simulink model "house_dynamics"  (R2015b)
settings: Solver=VariableStepAuto  StartTime=0.0  StopTime=len_sim*3600  RelTol=1e-3
values from neighbouring files (symbols this model uses):
  amb_CO = xlsread(filename,'Sheet1','X33')    [main_code.m]
  amb_CO2 = xlsread(filename,'Sheet1','X32')    [main_code.m]
  amb_PM = xlsread(filename,'Sheet1','X34')    [main_code.m]
  Cp_air = xlsread(filename,'Sheet1','X29')    [main_code.m]
  h_wall = xlsread(filename,'Sheet1','I30')    [main_code.m]
  k_door = door(1)    [main_code.m]
  k_floor = floor(1)    [main_code.m]
  k_roof_1 = roof_1(1)    [main_code.m]
  k_roof_2 = roof_2(1)    [main_code.m]
  k_roof_3 = roof_3(1)    [main_code.m]
  k_roof_4 = roof_4(1)    [main_code.m]
  k_roof_5 = roof_5(1)    [main_code.m]
  k_wall_a_1 = wall_a_1(1)    [main_code.m]
  k_wall_a_2 = wall_a_2(1)    [main_code.m]
  k_wall_a_3 = wall_a_3(1)    [main_code.m]
  k_wall_a_4 = wall_a_4(1)    [main_code.m]
  k_wall_a_5 = wall_a_5(1)    [main_code.m]
  k_wall_b_1 = wall_b_1(1)    [main_code.m]
  k_wall_b_2 = wall_b_2(1)    [main_code.m]
  k_wall_b_3 = wall_b_3(1)    [main_code.m]
  k_wall_b_4 = wall_b_4(1)    [main_code.m]
  k_wall_b_5 = wall_b_5(1)    [main_code.m]
  k_wall_c_1 = wall_c_1(1)    [main_code.m]
  k_wall_c_2 = wall_c_2(1)    [main_code.m]
  k_wall_c_4 = wall_c_4(1)    [main_code.m]
  k_wall_c_5 = wall_c_5(1)    [main_code.m]
  k_wall_d_1 = wall_d_1(1)    [main_code.m]
  k_wall_d_2 = wall_d_2(1)    [main_code.m]
  k_wall_d_3 = wall_d_3(1)    [main_code.m]
  k_wall_d_4 = wall_d_4(1)    [main_code.m]
  k_wall_d_5 = wall_d_5(1)    [main_code.m]
  k_window = window(1)    [main_code.m]
  l_wall = xlsread(filename,'Sheet1','I29')    [main_code.m]
  roof_c1 = alpha_roof_1/(t_roof_1*t_roof_1)    [main_code.m]
  roof_c2 = alpha_roof_2/(t_roof_2*t_roof_2)    [main_code.m]
  roof_c3 = alpha_roof_3/(t_roof_3*t_roof_3)    [main_code.m]
  roof_c4 = alpha_roof_4/(t_roof_4*t_roof_4)    [main_code.m]
  roof_c5 = alpha_roof_5/(t_roof_5*t_roof_5)    [main_code.m]
  roof_p1 = 4*t_roof_1*hb/k_roof_1    [main_code.m]
  roof_p2 = 4*t_roof_5*hinf/k_roof_5    [main_code.m]
  t_door = door(5)    [main_code.m]
  t_floor = floor(5)    [main_code.m]
  t_roof_1 = roof_1(5)    [main_code.m]
  t_roof_2 = roof_2(5)    [main_code.m]
  t_roof_3 = roof_3(5)    [main_code.m]
  t_roof_4 = roof_4(5)    [main_code.m]
  t_roof_5 = roof_5(5)    [main_code.m]
  t_wall_a_1 = wall_a_1(5)    [main_code.m]
  t_wall_a_2 = wall_a_2(5)    [main_code.m]
  t_wall_a_3 = wall_a_3(5)    [main_code.m]
  t_wall_a_4 = wall_a_4(5)    [main_code.m]
  t_wall_a_5 = wall_a_5(5)    [main_code.m]
  t_wall_b_1 = wall_b_1(5)    [main_code.m]
  t_wall_b_2 = wall_b_2(5)    [main_code.m]
  t_wall_b_3 = wall_b_3(5)    [main_code.m]
  t_wall_b_4 = wall_b_4(5)    [main_code.m]
  t_wall_b_5 = wall_b_5(5)    [main_code.m]
  t_wall_c_1 = wall_c_1(5)    [main_code.m]
  t_wall_c_2 = wall_c_2(5)    [main_code.m]
  t_wall_c_4 = wall_c_4(5)    [main_code.m]
  t_wall_c_5 = wall_c_5(5)    [main_code.m]
  t_wall_d_1 = wall_d_1(5)    [main_code.m]
  t_wall_d_2 = wall_d_2(5)    [main_code.m]
  t_wall_d_3 = wall_d_3(5)    [main_code.m]
  t_wall_d_4 = wall_d_4(5)    [main_code.m]
  t_wall_d_5 = wall_d_5(5)    [main_code.m]
  t_window = window(5)    [main_code.m]
  To = initial_room_temp    [main_code.m]
  w_wall = xlsread(filename,'Sheet1','I28')    [main_code.m]
settings Model: Creator=Sahil Desai  LastModifiedBy=Sahil Desai

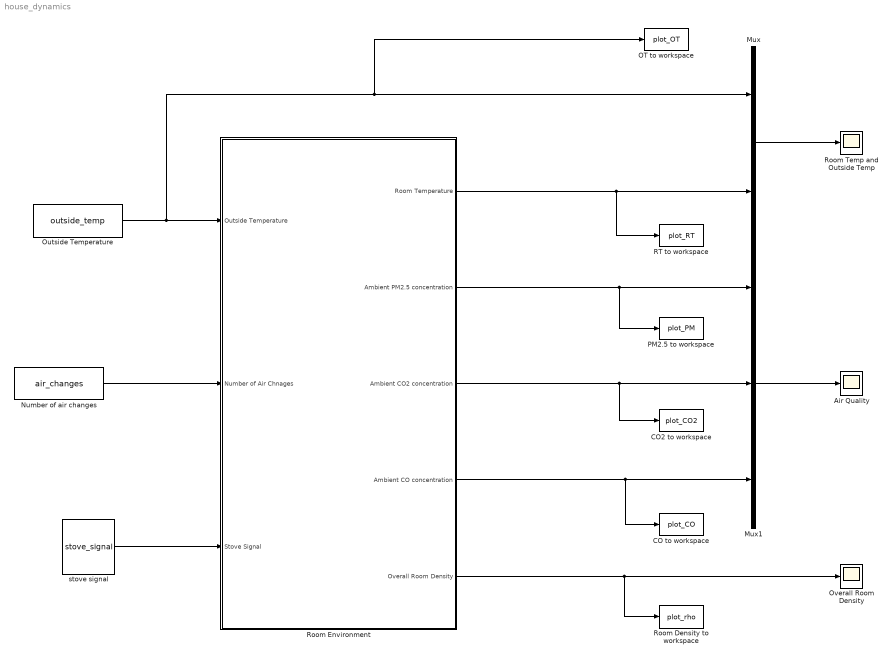
== system house_dynamics ==
  Air Quality : Scope
  CO to workspace : ToWorkspace  VariableName=plot_CO  SampleTime=-1
  CO2 to workspace : ToWorkspace  VariableName=plot_CO2  SampleTime=-1
  Mux : Mux  Inputs=2
  Mux1 : Mux  Inputs=3
  Number of air changes : FromWorkspace  VariableName=air_changes  SampleTime=0
  OT to workspace : ToWorkspace  VariableName=plot_OT  SampleTime=-1
  Outside Temperature : FromWorkspace  VariableName=outside_temp  SampleTime=0
  Overall Room Density : Scope
  PM2.5 to workspace : ToWorkspace  VariableName=plot_PM  SampleTime=-1
  RT to workspace : ToWorkspace  VariableName=plot_RT  SampleTime=-1
  Room Density to workspace : ToWorkspace  VariableName=plot_rho  SampleTime=-1
  Room Environment : Subsystem
  Room Temp and Outside Temp : Scope
  stove signal : FromWorkspace  VariableName=stove_signal  SampleTime=0
  wires:
  Number of air changes/1 -> Room Environment/2(Number of Air Chnages)
  stove signal/1 -> Room Environment/3(Stove Signal)
  Outside Temperature/1 -> OT to workspace/1, Mux/1, Room Environment/1(Outside Temperature)
  Mux/1 -> Room Temp and Outside Temp/1
  Mux1/1 -> Air Quality/1
  Room Environment/5(Overall Room Density) -> Room Density to workspace/1, Overall Room Density/1
  Room Environment/3(Ambient CO2 concentration) -> CO2 to workspace/1, Mux1/2
  Room Environment/2(Ambient PM2.5 concentration) -> PM2.5 to workspace/1, Mux1/1
  Room Environment/4(Ambient CO concentration) -> CO to workspace/1, Mux1/3
  Room Environment/1(Room Temperature) -> RT to workspace/1, Mux/2

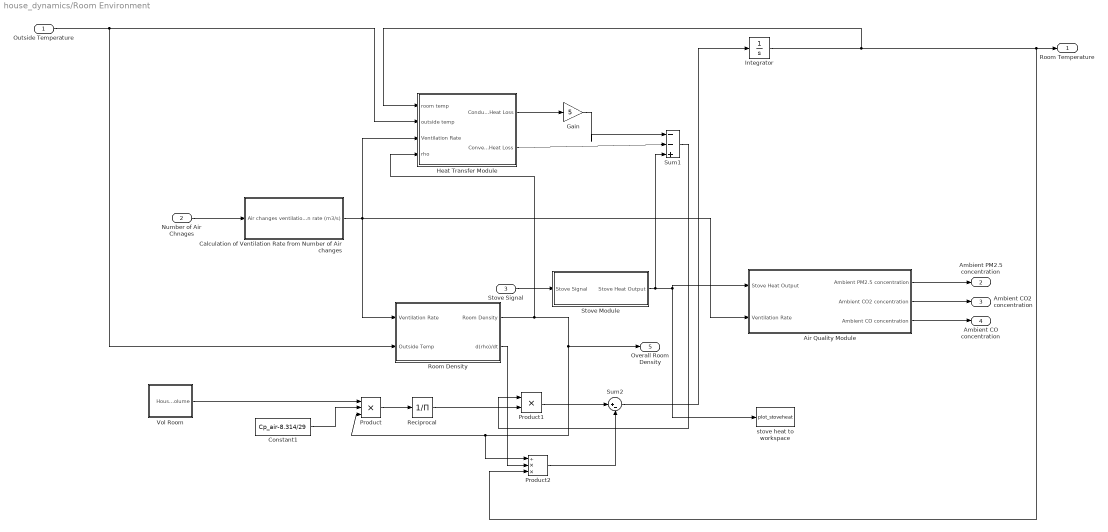
== system house_dynamics/Room Environment ==
  Outside Temperature : Inport
  Number of Air Chnages : Inport  Port=2
  Stove Signal : Inport  Port=3
  Air Quality Module : Subsystem
  Calculation of Ventilation Rate from Number of Air changes : Subsystem
  Constant1 : Constant  Value=Cp_air-8.314/29
  Gain : Gain  Gain=5
  Heat Transfer Module : Subsystem
  Integrator : Integrator  InitialCondition=5
  Product : Product  Inputs=3
  Product1 : Product
  Product2 : Product  Inputs=/**
  Reciprocal : Product  Inputs=/  SaturateOnIntegerOverflow=on  RndMeth=Zero
  Room Density : Subsystem
  Stove Module : Subsystem
  Sum1 : Sum  Inputs=|--+
  Sum2 : Sum  Inputs=|+-
  Vol Room : Subsystem
  stove heat to workspace : ToWorkspace  VariableName=plot_stoveheat  SampleTime=-1
  Room Temperature : Outport
  Ambient PM2.5 concentration : Outport  Port=2
  Ambient CO2 concentration : Outport  Port=3
  Ambient CO concentration : Outport  Port=4
  Overall Room Density : Outport  Port=5
  wires:
  Outside Temperature/1 -> Room Density/2(Outside Temp), Heat Transfer Module/2(outside temp)
  Integrator/1 -> Heat Transfer Module/1(room temp), Room Temperature/1, Product2/3
  Calculation of Ventilation Rate from Number of Air changes/1(ventilation rate (m3/s)) -> Room Density/1(Ventilation Rate), Air Quality Module/2(Ventilation Rate), Heat Transfer Module/3(Ventilation Rate)
  Number of Air Chnages/1 -> Calculation of Ventilation Rate from Number of Air changes/1(Air changes)
  Stove Signal/1 -> Stove Module/1(Stove Signal)
  Room Density/1(Room Density) -> Overall Room Density/1, Product2/1, Product/3, Heat Transfer Module/4(rho)
  Product/1 -> Reciprocal/1
  Reciprocal/1 -> Product1/2
  Sum1/1 -> Product1/1
  Product1/1 -> Sum2/1
  Room Density/2("d(rho)/dt ") -> Product2/2
  Product2/1 -> Sum2/2
  Sum2/1 -> Integrator/1
  Air Quality Module/3(Ambient CO concentration) -> Ambient CO concentration/1
  Air Quality Module/2(Ambient CO2 concentration) -> Ambient CO2 concentration/1
  Air Quality Module/1(Ambient PM2.5 concentration) -> Ambient PM2.5 concentration/1
  Constant1/1 -> Product/2
  Heat Transfer Module/2(Convective Heat Loss) -> Sum1/2
  Heat Transfer Module/1(Conductive Heat Loss) -> Gain/1
  Vol Room/1(House Volume) -> Product/1
  Gain/1 -> Sum1/1
  Stove Module/1(Stove Heat Output) -> stove heat to workspace/1, Air Quality Module/1(Stove Heat Output), Sum1/3

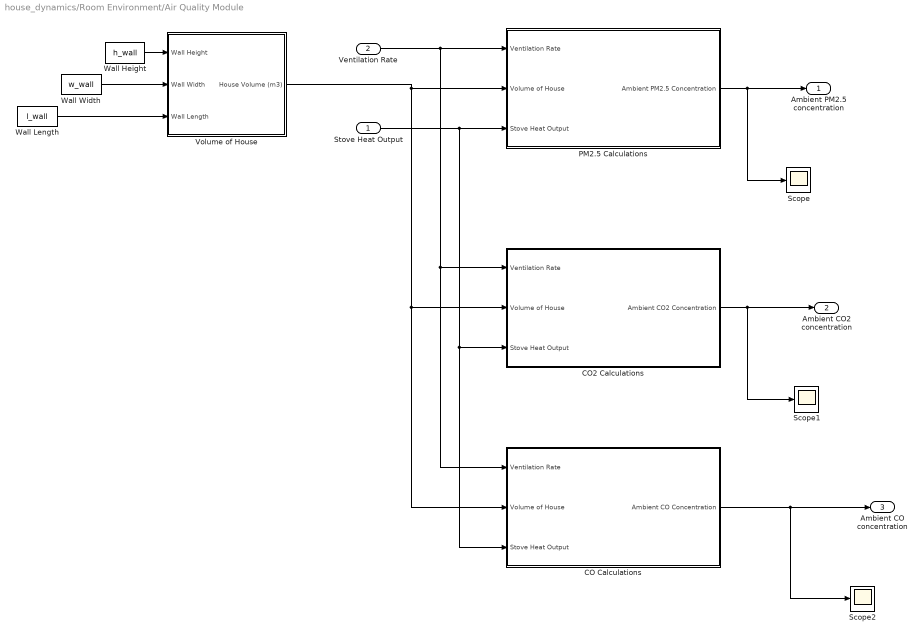
== system house_dynamics/Room Environment/Air Quality Module ==
  Stove Heat Output : Inport
  Ventilation Rate : Inport  Port=2
  CO Calculations : Subsystem
  CO2 Calculations : Subsystem
  PM2.5 Calculations : Subsystem
  Scope : Scope
  Scope1 : Scope
  Scope2 : Scope
  Volume of House : Subsystem  TreatAsAtomicUnit=on
  Wall Height : Constant  Value=h_wall
  Wall Length : Constant  Value=l_wall
  Wall Width : Constant  Value=w_wall
  Ambient PM2.5 concentration : Outport
  Ambient CO2 concentration : Outport  Port=2
  Ambient CO concentration : Outport  Port=3
  wires:
  Ventilation Rate/1 -> CO Calculations/1(Ventilation Rate), CO2 Calculations/1(Ventilation Rate), PM2.5 Calculations/1(Ventilation Rate)
  Stove Heat Output/1 -> CO Calculations/3(Stove Heat Output), CO2 Calculations/3(Stove Heat Output), PM2.5 Calculations/3(Stove Heat Output)
  PM2.5 Calculations/1(Ambient PM2.5 Concentration) -> Scope/1, Ambient PM2.5 concentration/1
  Volume of House/1(House Volume (m3)) -> CO Calculations/2(Volume of House), CO2 Calculations/2(Volume of House), PM2.5 Calculations/2(Volume of House)
  CO2 Calculations/1(Ambient CO2 Concentration) -> Ambient CO2 concentration/1, Scope1/1
  CO Calculations/1(Ambient CO Concentration) -> Scope2/1, Ambient CO concentration/1
  Wall Width/1 -> Volume of House/2(Wall Width)
  Wall Height/1 -> Volume of House/1(Wall Height)
  Wall Length/1 -> Volume of House/3(Wall Length)

== system house_dynamics/Room Environment/Calculation of Ventilation Rate from Number of Air changes ==
  Air changes : Inport
  Gain : Gain  Gain=1/3600
  Product1 : Product
  Volume of House : Subsystem  TreatAsAtomicUnit=on
  Wall Height : Constant  Value=h_wall
  Wall Length : Constant  Value=l_wall
  Wall Width : Constant  Value=w_wall
  ventilation rate (m3/s) : Outport
  wires:
  Gain/1 -> ventilation rate (m3/s)/1
  Product1/1 -> Gain/1
  Air changes/1 -> Product1/2
  Volume of House/1(House Volume (m3)) -> Product1/1
  Wall Width/1 -> Volume of House/2(Wall Width)
  Wall Height/1 -> Volume of House/1(Wall Height)
  Wall Length/1 -> Volume of House/3(Wall Length)

== system house_dynamics/Room Environment/Heat Transfer Module ==
  room temp : Inport
  outside temp : Inport  Port=2
  Ventilation Rate : Inport  Port=3
  rho : Inport  Port=4
  Conduction Heat Transfer : Subsystem
  Convective Heat Transfer : Subsystem
  Individual Roof Layer Temperatures : Scope
  Mux : Mux  Inputs=5
  Roof Heat Transfer1 : Subsystem
  Conductive Heat Loss : Outport
  Convective Heat Loss : Outport  Port=2
  wires:
  Ventilation Rate/1 -> Convective Heat Transfer/3(Ventilation Rate)
  outside temp/1 -> Roof Heat Transfer1/1(Outside Temperature), Convective Heat Transfer/1(Outside Temp), Conduction Heat Transfer/2(Outside Temperature)
  rho/1 -> Convective Heat Transfer/4(rho)
  room temp/1 -> Roof Heat Transfer1/2(Room Temperature), Convective Heat Transfer/2(room temp), Conduction Heat Transfer/1(Room Temperature)
  Conduction Heat Transfer/1("Conductive Heat Loss ") -> Conductive Heat Loss/1
  Convective Heat Transfer/1(Convective Heat Transfer) -> Convective Heat Loss/1
  Roof Heat Transfer1/5(Roof_T5) -> Mux/5
  Roof Heat Transfer1/4(Roof_T4) -> Mux/4
  Roof Heat Transfer1/3(Roof_T3) -> Mux/3
  Roof Heat Transfer1/2(Roof_T2) -> Mux/2
  Roof Heat Transfer1/1(Roof_T1) -> Mux/1
  Mux/1 -> Individual Roof Layer Temperatures/1

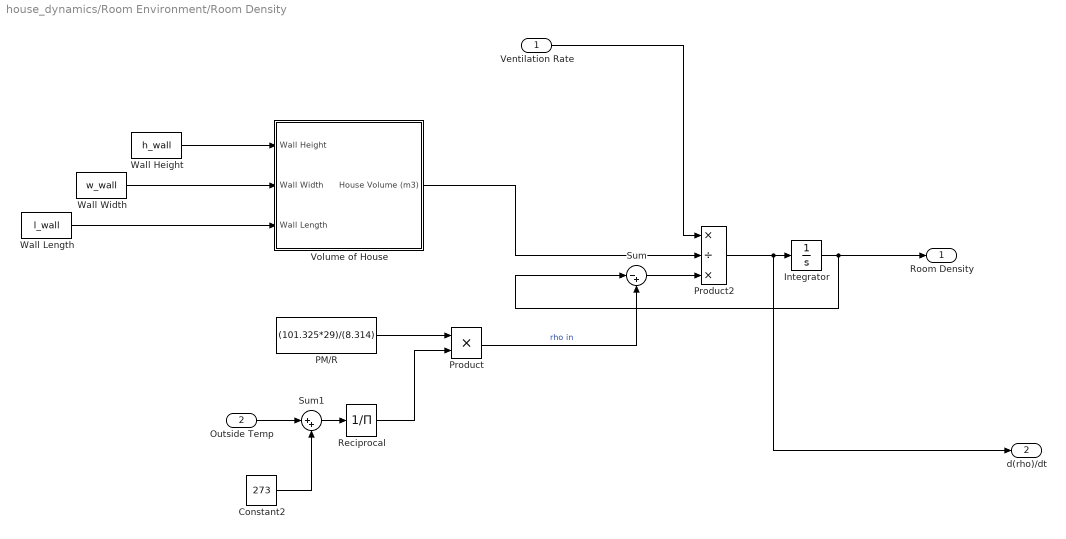
== system house_dynamics/Room Environment/Room Density ==
  Ventilation Rate : Inport
  Outside Temp : Inport  Port=2
  Constant2 : Constant  Value=273
  Integrator : Integrator  InitialCondition=1
  PM/R : Constant  Value=(101.325*29)/(8.314)
  Product : Product
  Product2 : Product  Inputs=*/*
  Reciprocal : Product  Inputs=/  SaturateOnIntegerOverflow=on  RndMeth=Zero
  Sum : Sum  Inputs=|-+
  Sum1 : Sum  Inputs=|++
  Volume of House : Subsystem  TreatAsAtomicUnit=on
  Wall Height : Constant  Value=h_wall
  Wall Length : Constant  Value=l_wall
  Wall Width : Constant  Value=w_wall
  Room Density : Outport
  "d(rho)/dt " : Outport  Port=2
  wires:
  Reciprocal/1 -> Product/2
  PM/R/1 -> Product/1
  Product/1 -> Sum/2  "rho in"
  Sum/1 -> Product2/3
  Product2/1 -> "d(rho)/dt "/1, Integrator/1
  Integrator/1 -> Sum/1, Room Density/1
  Outside Temp/1 -> Sum1/1
  Constant2/1 -> Sum1/2
  Sum1/1 -> Reciprocal/1
  Volume of House/1(House Volume (m3)) -> Product2/2
  Wall Width/1 -> Volume of House/2(Wall Width)
  Wall Height/1 -> Volume of House/1(Wall Height)
  Wall Length/1 -> Volume of House/3(Wall Length)
  Ventilation Rate/1 -> Product2/1

== system house_dynamics/Room Environment/Stove Module ==
  Stove Signal : Inport
  Stove Heat : Subsystem
  Stove Heat Output : Outport
  wires:
  Stove Signal/1 -> Stove Heat/1(Stove Signal)
  Stove Heat/1(Stove Heat Out) -> Stove Heat Output/1

== system house_dynamics/Room Environment/Vol Room ==
  Volume of House : Subsystem  TreatAsAtomicUnit=on
  Wall Height : Constant  Value=h_wall
  Wall Length : Constant  Value=l_wall
  Wall Width : Constant  Value=w_wall
  House Volume : Outport
  wires:
  Volume of House/1(House Volume (m3)) -> House Volume/1
  Wall Width/1 -> Volume of House/2(Wall Width)
  Wall Height/1 -> Volume of House/1(Wall Height)
  Wall Length/1 -> Volume of House/3(Wall Length)

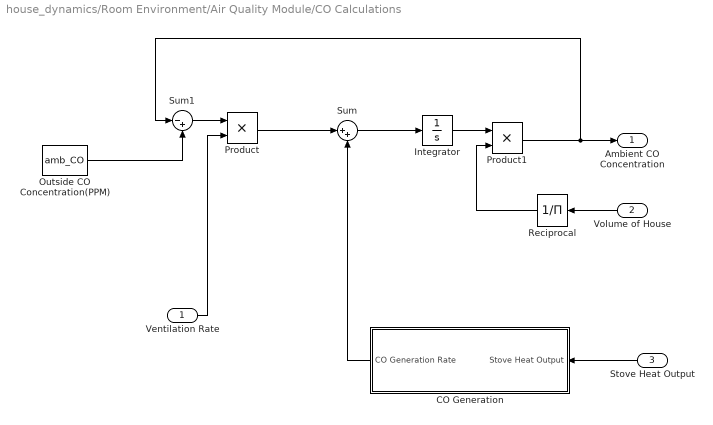
== system house_dynamics/Room Environment/Air Quality Module/CO Calculations ==
  Ventilation Rate : Inport
  Volume of House : Inport  Port=2
  Stove Heat Output : Inport  Port=3
  CO Generation : Subsystem
  Integrator : Integrator  InitialCondition=2
  Outside CO Concentration(PPM) : Constant  Value=amb_CO
  Product : Product
  Product1 : Product
  Reciprocal : Product  Inputs=/  SaturateOnIntegerOverflow=on  RndMeth=Zero
  Sum : Sum  Inputs=|++
  Sum1 : Sum  Inputs=|-+
  Ambient CO Concentration : Outport
  wires:
  Sum/1 -> Integrator/1
  Product/1 -> Sum/1
  CO Generation/1(CO Generation Rate) -> Sum/2
  Stove Heat Output/1 -> CO Generation/1(Stove Heat Output)
  Volume of House/1 -> Reciprocal/1
  Integrator/1 -> Product1/1
  Product1/1 -> Sum1/1, Ambient CO Concentration/1
  Reciprocal/1 -> Product1/2
  Sum1/1 -> Product/1
  Ventilation Rate/1 -> Product/2
  Outside CO Concentration(PPM)/1 -> Sum1/2

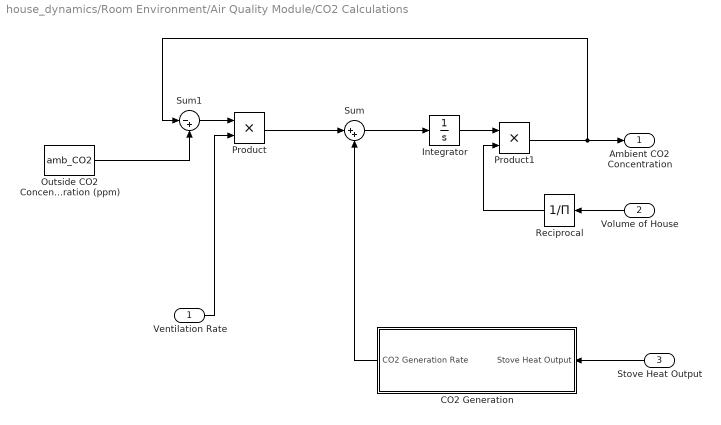
== system house_dynamics/Room Environment/Air Quality Module/CO2 Calculations ==
  Ventilation Rate : Inport
  Volume of House : Inport  Port=2
  Stove Heat Output : Inport  Port=3
  CO2 Generation : Subsystem
  Integrator : Integrator
  Outside CO2 Concentration (ppm) : Constant  Value=amb_CO2
  Product : Product
  Product1 : Product
  Reciprocal : Product  Inputs=/  SaturateOnIntegerOverflow=on  RndMeth=Zero
  Sum : Sum  Inputs=|++
  Sum1 : Sum  Inputs=|-+
  Ambient CO2 Concentration : Outport
  wires:
  Sum/1 -> Integrator/1
  Product/1 -> Sum/1
  CO2 Generation/1(CO2 Generation Rate) -> Sum/2
  Stove Heat Output/1 -> CO2 Generation/1(Stove Heat Output)
  Volume of House/1 -> Reciprocal/1
  Integrator/1 -> Product1/1
  Product1/1 -> Sum1/1, Ambient CO2 Concentration/1
  Reciprocal/1 -> Product1/2
  Sum1/1 -> Product/1
  Ventilation Rate/1 -> Product/2
  Outside CO2 Concentration (ppm)/1 -> Sum1/2

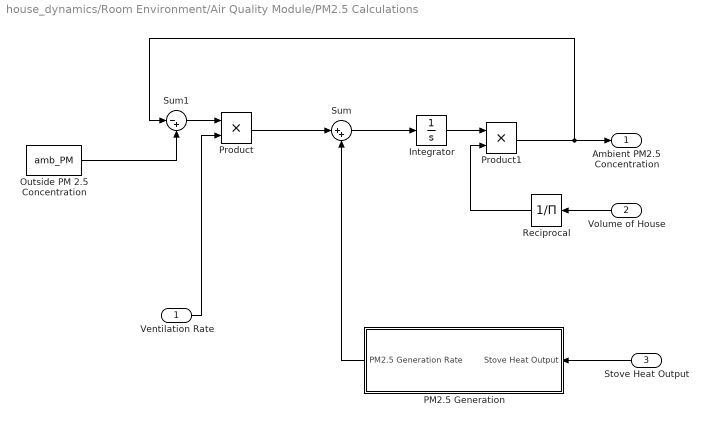
== system house_dynamics/Room Environment/Air Quality Module/PM2.5 Calculations ==
  Ventilation Rate : Inport
  Volume of House : Inport  Port=2
  Stove Heat Output : Inport  Port=3
  Integrator : Integrator
  Outside PM 2.5 Concentration : Constant  Value=amb_PM
  PM2.5 Generation : Subsystem
  Product : Product
  Product1 : Product
  Reciprocal : Product  Inputs=/  SaturateOnIntegerOverflow=on  RndMeth=Zero
  Sum : Sum  Inputs=|++
  Sum1 : Sum  Inputs=|-+
  Ambient PM2.5 Concentration : Outport
  wires:
  Sum/1 -> Integrator/1
  Product/1 -> Sum/1
  PM2.5 Generation/1(PM2.5 Generation Rate) -> Sum/2
  Stove Heat Output/1 -> PM2.5 Generation/1(Stove Heat Output)
  Volume of House/1 -> Reciprocal/1
  Integrator/1 -> Product1/1
  Product1/1 -> Sum1/1, Ambient PM2.5 Concentration/1
  Reciprocal/1 -> Product1/2
  Sum1/1 -> Product/1
  Ventilation Rate/1 -> Product/2
  Outside PM 2.5 Concentration/1 -> Sum1/2

== system house_dynamics/Room Environment/Air Quality Module/Volume of House ==
  Wall Height : Inport
  Wall Width : Inport  Port=2
  Wall Length : Inport  Port=3
  Product : Product  Inputs=3
  House Volume (m3) : Outport
  wires:
  Wall Height/1 -> Product/1
  Wall Width/1 -> Product/2
  Wall Length/1 -> Product/3
  Product/1 -> House Volume (m3)/1

== system house_dynamics/Room Environment/Calculation of Ventilation Rate from Number of Air changes/Volume of House ==
  Wall Height : Inport
  Wall Width : Inport  Port=2
  Wall Length : Inport  Port=3
  Product : Product  Inputs=3
  House Volume (m3) : Outport
  wires:
  Wall Height/1 -> Product/1
  Wall Width/1 -> Product/2
  Wall Length/1 -> Product/3
  Product/1 -> House Volume (m3)/1

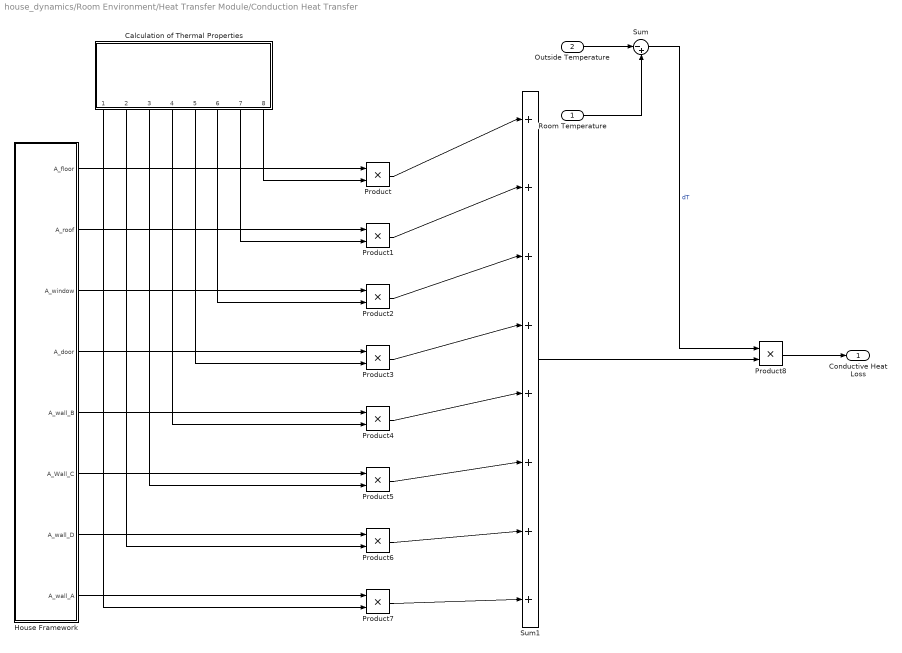
== system house_dynamics/Room Environment/Heat Transfer Module/Conduction Heat Transfer ==
  Room Temperature : Inport
  Outside Temperature : Inport  Port=2
  Calculation of Thermal Properties : Subsystem
  House Framework : Subsystem
  Product{,1..7} (8 alike) : Product  Inputs=**
  Product8 : Product
  Sum : Sum  Inputs=|-+
  Sum1 : Sum  Inputs=|++++++++
  "Conductive Heat Loss " : Outport
  wires:
  House Framework/1(A_floor) -> Product/1
  House Framework/2(A_roof) -> Product1/1
  House Framework/3(A_window) -> Product2/1
  House Framework/4(A_door) -> Product3/1
  House Framework/5(A_wall_B) -> Product4/1
  House Framework/6(A_Wall_C) -> Product5/1
  House Framework/7(A_wall_D) -> Product6/1
  House Framework/8(A_wall_A) -> Product7/1
  Product/1 -> Sum1/1
  Product1/1 -> Sum1/2
  Product2/1 -> Sum1/3
  Product3/1 -> Sum1/4
  Product4/1 -> Sum1/5
  Product5/1 -> Sum1/6
  Product6/1 -> Sum1/7
  Product7/1 -> Sum1/8
  Sum1/1 -> Product8/2
  Sum/1 -> Product8/1  "dT"
  Outside Temperature/1 -> Sum/1
  Room Temperature/1 -> Sum/2
  Product8/1 -> "Conductive Heat Loss "/1
  Calculation of Thermal Properties/8(U_eq_floor) -> Product/2
  Calculation of Thermal Properties/7(U_eq_roof) -> Product1/2
  Calculation of Thermal Properties/6(U_eq_window) -> Product2/2
  Calculation of Thermal Properties/5(U_eq_door) -> Product3/2
  Calculation of Thermal Properties/1(U_eq_wall_A) -> Product7/2
  Calculation of Thermal Properties/2(U_eq_wall_D) -> Product6/2
  Calculation of Thermal Properties/3(U_eq_wall_C) -> Product5/2
  Calculation of Thermal Properties/4(U_eq_wall_B) -> Product4/2

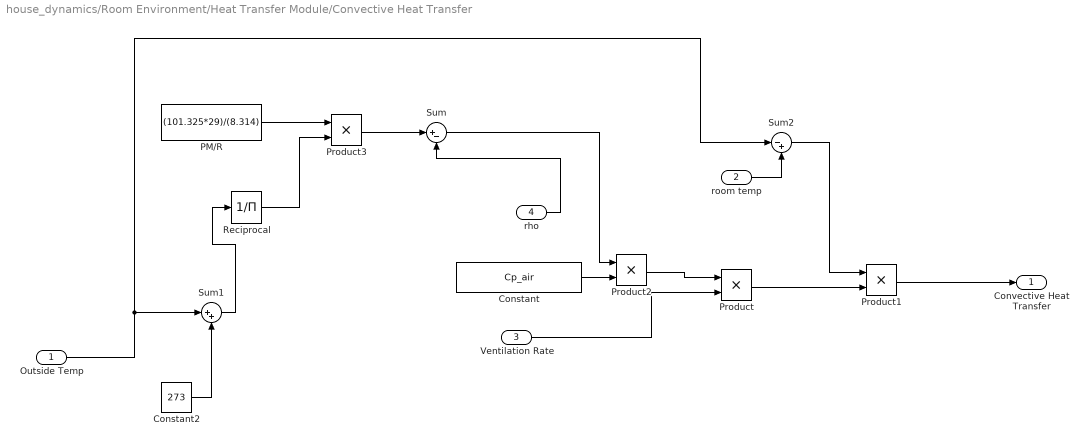
== system house_dynamics/Room Environment/Heat Transfer Module/Convective Heat Transfer ==
  Outside Temp : Inport
  room temp : Inport  Port=2
  Ventilation Rate : Inport  Port=3
  rho : Inport  Port=4
  Constant : Constant  Value=Cp_air
  Constant2 : Constant  Value=273
  PM/R : Constant  Value=(101.325*29)/(8.314)
  Product{,1..3} (4 alike) : Product
  Reciprocal : Product  Inputs=/  SaturateOnIntegerOverflow=on  RndMeth=Zero
  Sum : Sum  Inputs=|+-
  Sum1 : Sum  Inputs=|++
  Sum2 : Sum  Inputs=|-+
  Convective Heat Transfer : Outport
  wires:
  Ventilation Rate/1 -> Product/2
  Product/1 -> Product1/2
  Product1/1 -> Convective Heat Transfer/1
  Constant/1 -> Product2/2
  Product2/1 -> Product/1
  rho/1 -> Sum/2
  Reciprocal/1 -> Product3/2
  PM/R/1 -> Product3/1
  Outside Temp/1 -> Sum2/1, Sum1/1
  Constant2/1 -> Sum1/2
  Sum1/1 -> Reciprocal/1
  Product3/1 -> Sum/1
  Sum/1 -> Product2/1
  Sum2/1 -> Product1/1
  room temp/1 -> Sum2/2

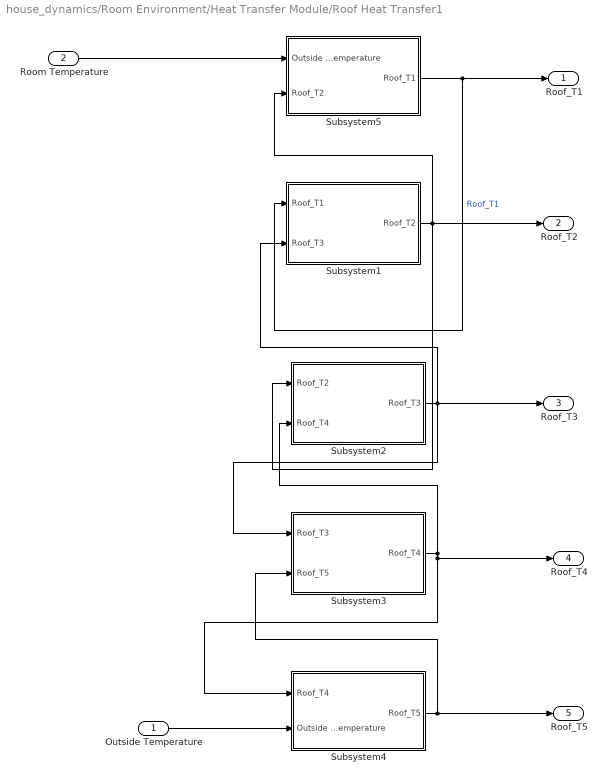
== system house_dynamics/Room Environment/Heat Transfer Module/Roof Heat Transfer1 ==
  Outside Temperature : Inport
  Room Temperature : Inport  Port=2
  Subsystem1 : Subsystem
  Subsystem2 : Subsystem
  Subsystem3 : Subsystem
  Subsystem4 : Subsystem
  Subsystem5 : Subsystem
  Roof_T1 : Outport
  Roof_T2 : Outport  Port=2
  Roof_T3 : Outport  Port=3
  Roof_T4 : Outport  Port=4
  Roof_T5 : Outport  Port=5
  wires:
  Room Temperature/1 -> Subsystem5/1(Outside Temperature)
  Subsystem5/1(Roof_T1) -> Roof_T1/1, Subsystem1/1(Roof_T1)  "Roof_T1"
  Subsystem1/1(Roof_T2) -> Roof_T2/1, Subsystem5/2(Roof_T2), Subsystem2/1(Roof_T2)
  Subsystem2/1(Roof_T3) -> Subsystem3/1(Roof_T3), Roof_T3/1, Subsystem1/2(Roof_T3)
  Subsystem3/1(Roof_T4) -> Roof_T4/1, Subsystem4/1(Roof_T4), Subsystem2/2(Roof_T4)
  Outside Temperature/1 -> Subsystem4/2(Outside Temperature)
  Subsystem4/1(Roof_T5) -> Roof_T5/1, Subsystem3/2(Roof_T5)

== system house_dynamics/Room Environment/Room Density/Volume of House ==
  Wall Height : Inport
  Wall Width : Inport  Port=2
  Wall Length : Inport  Port=3
  Product : Product  Inputs=3
  House Volume (m3) : Outport
  wires:
  Wall Height/1 -> Product/1
  Wall Width/1 -> Product/2
  Wall Length/1 -> Product/3
  Product/1 -> House Volume (m3)/1

== system house_dynamics/Room Environment/Stove Module/Stove Heat ==
  Stove Signal : Inport
  Product1 : Product
  stove firepower : FromWorkspace  VariableName=fire_power  SampleTime=0
  Stove Heat Out : Outport
  wires:
  Product1/1 -> Stove Heat Out/1
  Stove Signal/1 -> Product1/1
  stove firepower/1 -> Product1/2

== system house_dynamics/Room Environment/Vol Room/Volume of House ==
  Wall Height : Inport
  Wall Width : Inport  Port=2
  Wall Length : Inport  Port=3
  Product : Product  Inputs=3
  House Volume (m3) : Outport
  wires:
  Wall Height/1 -> Product/1
  Wall Width/1 -> Product/2
  Wall Length/1 -> Product/3
  Product/1 -> House Volume (m3)/1

== system house_dynamics/Room Environment/Air Quality Module/CO Calculations/CO Generation ==
  Stove Heat Output : Inport
  MATLAB Function : MATLAB Function  TreatAsAtomicUnit=on
  CO Generation Rate : Outport
  wires:
  Stove Heat Output/1 -> MATLAB Function/1(u)
  MATLAB Function/1(y) -> CO Generation Rate/1

== system house_dynamics/Room Environment/Air Quality Module/CO2 Calculations/CO2 Generation ==
  Stove Heat Output : Inport
  MATLAB Function : MATLAB Function  TreatAsAtomicUnit=on
  CO2 Generation Rate : Outport
  wires:
  Stove Heat Output/1 -> MATLAB Function/1(u)
  MATLAB Function/1(y) -> CO2 Generation Rate/1

== system house_dynamics/Room Environment/Air Quality Module/PM2.5 Calculations/PM2.5 Generation ==
  Stove Heat Output : Inport
  MATLAB Function : MATLAB Function  TreatAsAtomicUnit=on
  PM2.5 Generation Rate : Outport
  wires:
  Stove Heat Output/1 -> MATLAB Function/1(u)
  MATLAB Function/1(y) -> PM2.5 Generation Rate/1

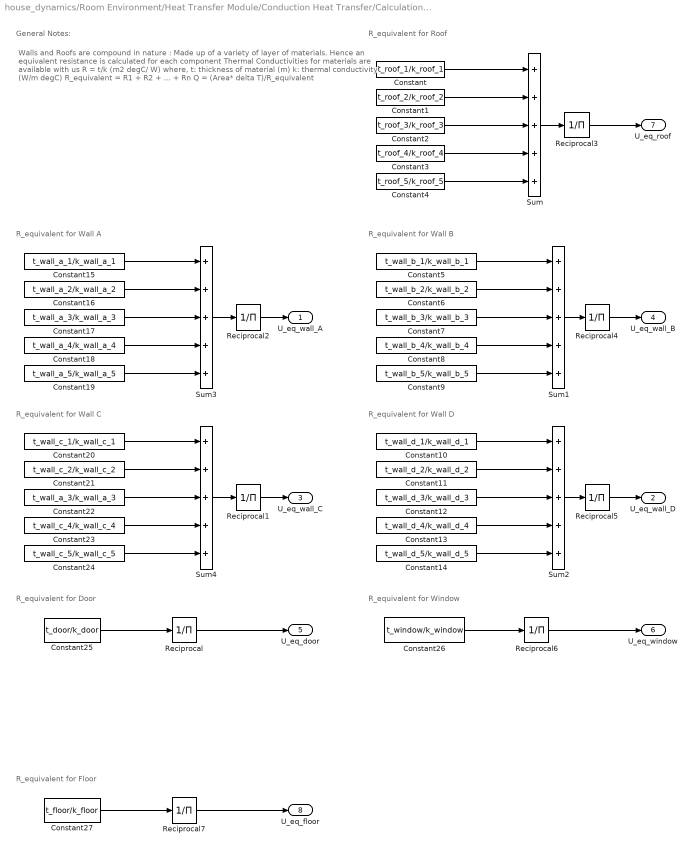
== system house_dynamics/Room Environment/Heat Transfer Module/Conduction Heat Transfer/Calculation of Thermal Properties ==
  note: General Notes:
  note: R_equivalent for Roof
  note: Walls and Roofs are compound in nature : Made up of a variety of layer of materials.
      |
      | Hence an equivalent resistance is calculated for each component
      |
      | Thermal Conductivities for materials are available with us
      |
      | R = t/k (m2 degC/ W)
      | where,
      | t: thickness of material (m)
      | k: thermal conductivity (W/m degC)
      |
      | R_equivalent = R1 + R2 + ... + Rn
      |
      | Q = (Area* delta T)/R_equivalent
  note: R_equivalent for Wall B
  note: R_equivalent for Wall D
  note: R_equivalent for Wall A
  note: R_equivalent for Wall C
  note: R_equivalent for Door
  note: R_equivalent for Window
  note: R_equivalent for Floor
  Constant : Constant  Value=t_roof_1/k_roof_1
  Constant1 : Constant  Value=t_roof_2/k_roof_2
  Constant10 : Constant  Value=t_wall_d_1/k_wall_d_1
  Constant11 : Constant  Value=t_wall_d_2/k_wall_d_2
  Constant12 : Constant  Value=t_wall_d_3/k_wall_d_3
  Constant13 : Constant  Value=t_wall_d_4/k_wall_d_4
  Constant14 : Constant  Value=t_wall_d_5/k_wall_d_5
  Constant15 : Constant  Value=t_wall_a_1/k_wall_a_1
  Constant16 : Constant  Value=t_wall_a_2/k_wall_a_2
  Constant17 : Constant  Value=t_wall_a_3/k_wall_a_3
  Constant18 : Constant  Value=t_wall_a_4/k_wall_a_4
  Constant19 : Constant  Value=t_wall_a_5/k_wall_a_5
  Constant2 : Constant  Value=t_roof_3/k_roof_3
  Constant20 : Constant  Value=t_wall_c_1/k_wall_c_1
  Constant21 : Constant  Value=t_wall_c_2/k_wall_c_2
  Constant22 : Constant  Value=t_wall_a_3/k_wall_a_3
  Constant23 : Constant  Value=t_wall_c_4/k_wall_c_4
  Constant24 : Constant  Value=t_wall_c_5/k_wall_c_5
  Constant25 : Constant  Value=t_door/k_door
  Constant26 : Constant  Value=t_window/k_window
  Constant27 : Constant  Value=t_floor/k_floor
  Constant3 : Constant  Value=t_roof_4/k_roof_4
  Constant4 : Constant  Value=t_roof_5/k_roof_5
  Constant5 : Constant  Value=t_wall_b_1/k_wall_b_1
  Constant6 : Constant  Value=t_wall_b_2/k_wall_b_2
  Constant7 : Constant  Value=t_wall_b_3/k_wall_b_3
  Constant8 : Constant  Value=t_wall_b_4/k_wall_b_4
  Constant9 : Constant  Value=t_wall_b_5/k_wall_b_5
  Reciprocal{,1..7} (8 alike) : Product  Inputs=/  SaturateOnIntegerOverflow=on  RndMeth=Zero
  Sum{,1..4} (5 alike) : Sum  Inputs=5
  U_eq_wall_A : Outport
  U_eq_wall_D : Outport  Port=2
  U_eq_wall_C : Outport  Port=3
  U_eq_wall_B : Outport  Port=4
  U_eq_door : Outport  Port=5
  U_eq_window : Outport  Port=6
  U_eq_roof : Outport  Port=7
  U_eq_floor : Outport  Port=8
  wires:
  Constant/1 -> Sum/1
  Constant1/1 -> Sum/2
  Constant2/1 -> Sum/3
  Constant3/1 -> Sum/4
  Constant4/1 -> Sum/5
  Sum/1 -> Reciprocal3/1
  Constant5/1 -> Sum1/1
  Sum1/1 -> Reciprocal4/1
  Constant6/1 -> Sum1/2
  Constant7/1 -> Sum1/3
  Constant8/1 -> Sum1/4
  Constant9/1 -> Sum1/5
  Constant10/1 -> Sum2/1
  Sum2/1 -> Reciprocal5/1
  Constant11/1 -> Sum2/2
  Constant12/1 -> Sum2/3
  Constant13/1 -> Sum2/4
  Constant14/1 -> Sum2/5
  Constant15/1 -> Sum3/1
  Sum3/1 -> Reciprocal2/1
  Constant16/1 -> Sum3/2
  Constant17/1 -> Sum3/3
  Constant18/1 -> Sum3/4
  Constant19/1 -> Sum3/5
  Constant20/1 -> Sum4/1
  Sum4/1 -> Reciprocal1/1
  Constant21/1 -> Sum4/2
  Constant22/1 -> Sum4/3
  Constant23/1 -> Sum4/4
  Constant24/1 -> Sum4/5
  Constant25/1 -> Reciprocal/1
  Constant26/1 -> Reciprocal6/1
  Constant27/1 -> Reciprocal7/1
  Reciprocal/1 -> U_eq_door/1
  Reciprocal1/1 -> U_eq_wall_C/1
  Reciprocal2/1 -> U_eq_wall_A/1
  Reciprocal3/1 -> U_eq_roof/1
  Reciprocal4/1 -> U_eq_wall_B/1
  Reciprocal5/1 -> U_eq_wall_D/1
  Reciprocal6/1 -> U_eq_window/1
  Reciprocal7/1 -> U_eq_floor/1

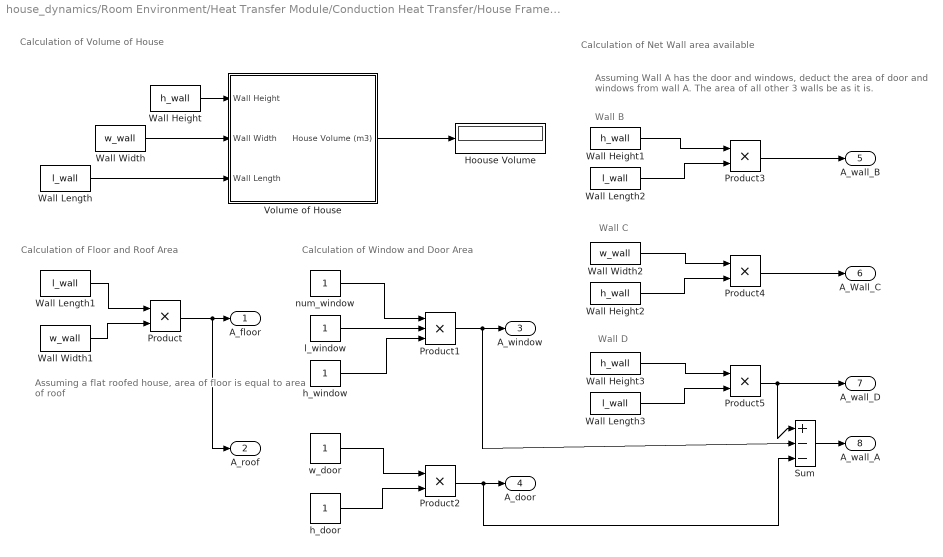
== system house_dynamics/Room Environment/Heat Transfer Module/Conduction Heat Transfer/House Framework ==
  note: Wall D
  note: Wall C
  note: Wall B
  note: Assuming Wall A has the door and windows, deduct the area of door
      | and windows from wall A. The area of all other 3 walls be as it is.
  note: Calculation of Net Wall area available
  note: Assuming a flat roofed house, area of  floor is equal
      | to area of roof
  note: Calculation of Floor and Roof Area
  note: Calculation of Volume of House
  note: Calculation of Window and Door Area
  "     num_window" : Constant
  Hoouse Volume : Display
  Product{,2..5} (5 alike) : Product
  Product1 : Product  Inputs=3
  Sum : Sum  Inputs=|+--
  Volume of House : Subsystem  TreatAsAtomicUnit=on
  Wall Height{,1..3} (4 alike) : Constant  Value=h_wall
  Wall Length{,1..3} (4 alike) : Constant  Value=l_wall
  Wall Width : Constant  Value=w_wall
  Wall Width1 : Constant  Value=w_wall
  Wall Width2 : Constant  Value=w_wall
  h_door : Constant
  h_window : Constant
  l_window : Constant
  w_door : Constant
  A_floor : Outport
  A_roof : Outport  Port=2
  A_window : Outport  Port=3
  A_door : Outport  Port=4
  A_wall_B : Outport  Port=5
  A_Wall_C : Outport  Port=6
  A_wall_D : Outport  Port=7
  A_wall_A : Outport  Port=8
  wires:
  Wall Width/1 -> Volume of House/2(Wall Width)
  Wall Height/1 -> Volume of House/1(Wall Height)
  Wall Length/1 -> Volume of House/3(Wall Length)
  Wall Length1/1 -> Product/1
  Wall Width1/1 -> Product/2
  Product/1 -> A_roof/1, A_floor/1
  Product1/1 -> A_window/1, Sum/2
  l_window/1 -> Product1/2
  "     num_window"/1 -> Product1/1
  h_window/1 -> Product1/3
  Product2/1 -> A_door/1, Sum/3
  w_door/1 -> Product2/1
  h_door/1 -> Product2/2
  Product3/1 -> A_wall_B/1
  Product4/1 -> A_Wall_C/1
  Product5/1 -> A_wall_D/1, Sum/1
  Wall Height1/1 -> Product3/1
  Wall Length2/1 -> Product3/2
  Wall Width2/1 -> Product4/1
  Wall Height2/1 -> Product4/2
  Wall Height3/1 -> Product5/1
  Wall Length3/1 -> Product5/2
  Sum/1 -> A_wall_A/1
  Volume of House/1(House Volume (m3)) -> Hoouse Volume/1

== system house_dynamics/Room Environment/Heat Transfer Module/Roof Heat Transfer1/Subsystem1 ==
  Roof_T1 : Inport
  Roof_T3 : Inport  Port=2
  Gain : Gain  Gain=0.5
  Gain1 : Gain  Gain=roof_c2
  Gain2 : Gain  Gain=0.5
  Gain3 : Gain  Gain=-1
  Integrator1 : Integrator  InitialCondition=To
  Sum1 : Sum  Inputs=|+++
  Roof_T2 : Outport
  wires:
  Gain1/1 -> Integrator1/1
  Sum1/1 -> Gain1/1
  Integrator1/1 -> Gain3/1, Roof_T2/1
  Roof_T3/1 -> Gain/1
  Gain/1 -> Sum1/2
  Roof_T1/1 -> Gain2/1
  Gain2/1 -> Sum1/1
  Gain3/1 -> Sum1/3

== system house_dynamics/Room Environment/Heat Transfer Module/Roof Heat Transfer1/Subsystem2 ==
  Roof_T2 : Inport
  Roof_T4 : Inport  Port=2
  Gain : Gain  Gain=0.5
  Gain1 : Gain  Gain=roof_c3
  Gain2 : Gain  Gain=0.5
  Gain3 : Gain  Gain=-1
  Integrator1 : Integrator  InitialCondition=To
  Sum1 : Sum  Inputs=|+++
  Roof_T3 : Outport
  wires:
  Gain1/1 -> Integrator1/1
  Sum1/1 -> Gain1/1
  Integrator1/1 -> Gain3/1, Roof_T3/1
  Roof_T2/1 -> Gain/1
  Gain/1 -> Sum1/2
  Roof_T4/1 -> Gain2/1
  Gain2/1 -> Sum1/1
  Gain3/1 -> Sum1/3

== system house_dynamics/Room Environment/Heat Transfer Module/Roof Heat Transfer1/Subsystem3 ==
  Roof_T3 : Inport
  Roof_T5 : Inport  Port=2
  Gain : Gain  Gain=0.5
  Gain1 : Gain  Gain=roof_c4
  Gain2 : Gain  Gain=0.5
  Gain3 : Gain  Gain=-1
  Integrator1 : Integrator  InitialCondition=To
  Sum1 : Sum  Inputs=|+++
  Roof_T4 : Outport
  wires:
  Gain1/1 -> Integrator1/1
  Sum1/1 -> Gain1/1
  Integrator1/1 -> Gain3/1, Roof_T4/1
  Roof_T3/1 -> Gain/1
  Gain/1 -> Sum1/2
  Roof_T5/1 -> Gain2/1
  Gain2/1 -> Sum1/1
  Gain3/1 -> Sum1/3

== system house_dynamics/Room Environment/Heat Transfer Module/Roof Heat Transfer1/Subsystem4 ==
  Roof_T4 : Inport
  Outside Temperature : Inport  Port=2
  Gain : Gain  Gain=roof_c5
  Gain1 : Gain  Gain=roof_p2
  Gain5 : Gain  Gain=1/(roof_p2+2)
  Gain6 : Gain  Gain=-1.5
  Gain7 : Gain  Gain=0.5
  Integrator : Integrator  InitialCondition=To
  Sum : Sum  Inputs=|+++
  Sum5 : Sum  Inputs=|+++
  Roof_T5 : Outport
  wires:
  Integrator/1 -> Sum5/1, Roof_T5/1, Gain6/1  "T1"
  Roof_T4/1 -> Gain7/1, Sum5/3  "T4"
  Gain/1 -> Integrator/1
  Sum/1 -> Gain/1
  Outside Temperature/1 -> Gain1/1
  Gain1/1 -> Sum5/2
  Sum5/1 -> Gain5/1  "T6_s"
  Gain6/1 -> Sum/3
  Gain7/1 -> Sum/2
  Gain5/1 -> Sum/1

== system house_dynamics/Room Environment/Heat Transfer Module/Roof Heat Transfer1/Subsystem5 ==
  Outside Temperature : Inport
  Roof_T2 : Inport  Port=2
  Gain : Gain  Gain=roof_c1
  Gain1 : Gain  Gain=roof_p1
  Gain5 : Gain  Gain=1/(roof_p1+2)
  Gain6 : Gain  Gain=-1.5
  Gain7 : Gain  Gain=0.5
  Integrator : Integrator  InitialCondition=To
  Sum : Sum  Inputs=|+++
  Sum5 : Sum  Inputs=|+++
  Roof_T1 : Outport
  wires:
  Integrator/1 -> Sum5/1, Roof_T1/1, Gain6/1  "T1"
  Roof_T2/1 -> Gain7/1, Sum5/3  "T4"
  Gain/1 -> Integrator/1
  Sum/1 -> Gain/1
  Outside Temperature/1 -> Gain1/1
  Gain1/1 -> Sum5/2
  Sum5/1 -> Gain5/1  "T1_s"
  Gain6/1 -> Sum/3
  Gain7/1 -> Sum/2
  Gain5/1 -> Sum/1

== system house_dynamics/Room Environment/Heat Transfer Module/Conduction Heat Transfer/House Framework/Volume of House ==
  Wall Height : Inport
  Wall Width : Inport  Port=2
  Wall Length : Inport  Port=3
  Product : Product  Inputs=3
  House Volume (m3) : Outport
  wires:
  Wall Height/1 -> Product/1
  Wall Width/1 -> Product/2
  Wall Length/1 -> Product/3
  Product/1 -> House Volume (m3)/1

== matlab function house_dynamics/Room Environment/Air Quality Module/CO Calculations/CO Generation/MATLAB Function ==
  data: u input; y output
function y = fcn(u)


y = (4.08*10^-5)*u;

== matlab function house_dynamics/Room Environment/Air Quality Module/CO2 Calculations/CO2 Generation/MATLAB Function ==
  data: u input; y output
function y = fcn(u)


y = (2*10^-5)*u;

== matlab function house_dynamics/Room Environment/Air Quality Module/PM2.5 Calculations/PM2.5 Generation/MATLAB Function ==
  data: u input; y output
function y = fcn(u)


y = (2*10^-5)*u;
